simulink model "Aim_23__Monocopter_Testing"  (R2023b)
settings: Solver=ode23t  StartTime=0.0  StopTime=10  MaxStep=1e-3  RelTol=1e-3  AbsTol=1e-3
values from neighbouring files (symbols this model uses):
  air_rho = 1.225    [Aim_23_inherited_params.mat]
  battery_capacity = 22.8    [Aim_23_inherited_params.mat]
  CDO = 10.25    [Aim_23_inherited_params.mat]
  drag_linear = 0.002    [Aim_23_inherited_params.mat]
  drag_quad = 0.005    [Aim_23_inherited_params.mat]
  filtD_motor = 100    [Aim_23_inherited_params.mat]
  filtSpd_motor = 0.001    [Aim_23_inherited_params.mat]
  flap_radius = 0.05312    [Aim_23_inherited_params.mat]
  flap_surface_area = 0.025    [Aim_23_inherited_params.mat]
  kd_motor = 0    [Aim_23_inherited_params.mat]
  ki_motor = 0.00045    [Aim_23_inherited_params.mat]
  klinear = 0.03    [Aim_23_inherited_params.mat]
  kquad = 0.025    [Aim_23_inherited_params.mat]
  limit_motor = 0.25    [Aim_23_inherited_params.mat]
  monoco_mass = 160    [Aim_23_inherited_params.mat]
  monoco_prop =     [Aim_23_inherited_params.mat]
  monoco_radius = 0.61    [Aim_23_inherited_params.mat]
  monoco_wing =     [Aim_23_inherited_params.mat]
  monoco_wing_area = 0.239    [Aim_23_inherited_params.mat]
  waypoints = [-2 -2 0.14 -2 -2 6 0 0 6 2 0 6 ... (15 elements, 3x5)]    [Aim_23_inherited_params.mat]
undefined symbols (not defined in the file or in its folder): X, Y, Z
libraries: sm_lib x97, nesl_utility x38, slpidlib x18, fl_lib x12, sdl_lib x3, simulink x2, simulink_extras x1, batteryecm_lib x1, ee_lib x1
(part 2 of 7)

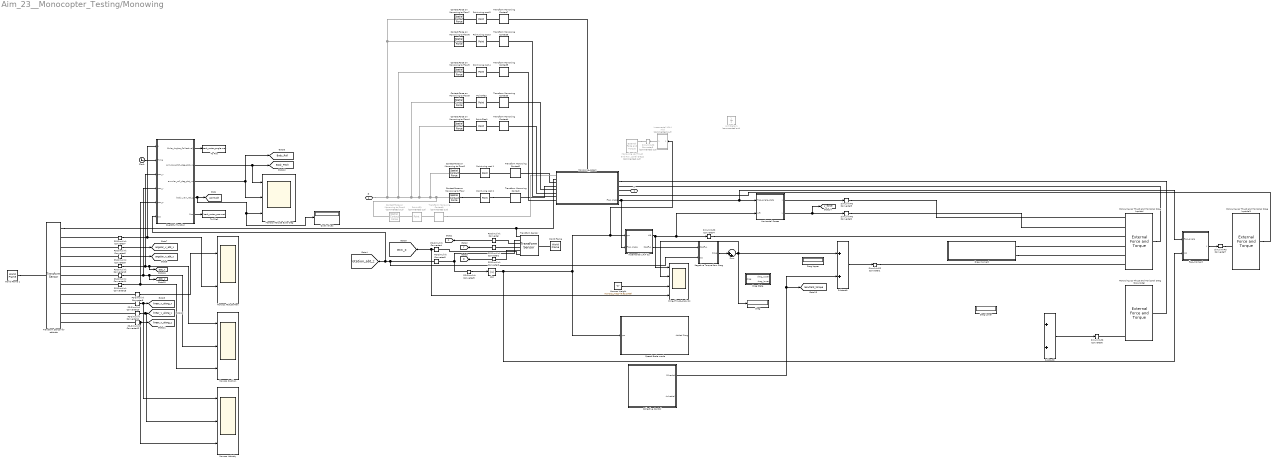
== system Aim_23__Monocopter_Testing/Monowing ==
  Abs : Abs  SaturateOnIntegerOverflow=off
  Clock : Clock
  Collective Control : Subsystem
  Contact Force on Monowing to Floor{,2..7} (7 alike) : sm_lib/Forces and Torques/Spatial Contact Force  SenseContactBaseRotation=off  SenseContactBaseTranslation=off  CoefficientOfDynamicFriction=0  CoefficientOfStaticFriction=0  NormalDamping=pkgGrndDamp  NormalDampingUnits=N/(m/s)  SenseContactSignal=off  NormalStiffness=pkgGrndStiff  NormalStiffnessUnits=N/m  FrictionalCriticalVelocity=1e-2  FrictionalCriticalVelocityUnits=m/s  ZeroCrossDetectContactStartAndEnd=off  SenseContactFollowerRotation=off  SenseContactFollowerTranslation=off  FrictionType=SmoothStickSlip  SenseFrictionalForceMagnitude=off  SenseNormalForceMagnitude=off  NormalForceType=SmoothSpringDamper  SenseNormalVelocity=off  SensePenetrationDepth=off  SenseSeparationDistance=off  SenseTangentialVelocity=off  NormalTransitionRegionWidth=pkgGrndTransW  NormalTransitionRegionWidthUnits=m
  Contact Force on Monowing to Floor1 : sm_lib/Forces and Torques/Spatial Contact Force  Commented=on  SenseContactBaseRotation=off  SenseContactBaseTranslation=off  CoefficientOfDynamicFriction=0  CoefficientOfStaticFriction=0  NormalDamping=pkgGrndDamp  NormalDampingUnits=N/(m/s)  SenseContactSignal=off  NormalStiffness=pkgGrndStiff  NormalStiffnessUnits=N/m  FrictionalCriticalVelocity=1e-2  FrictionalCriticalVelocityUnits=m/s  ZeroCrossDetectContactStartAndEnd=off  SenseContactFollowerRotation=off  SenseContactFollowerTranslation=off  FrictionType=SmoothStickSlip  SenseFrictionalForceMagnitude=off  SenseNormalForceMagnitude=off  NormalForceType=SmoothSpringDamper  SenseNormalVelocity=off  SensePenetrationDepth=off  SenseSeparationDistance=off  SenseTangentialVelocity=off  NormalTransitionRegionWidth=pkgGrndTransW  NormalTransitionRegionWidthUnits=m
  Drag : Display
  Drag Lower : Display
  Drag State : Subsystem
  Drag Upper : Display
  Drag moment : Subsystem
  Horizontal Forces : Subsystem
  Incremental Lift 4 mid : Subsystem  Commented=on
  Incremental Lift 4 tip : Subsystem
  Monoco Attitude Euler Deg : Scope  NumInputPorts=3
  Monoco Attitude Raw : Scope  NumInputPorts=2
  Monoco Position : Scope  NumInputPorts=3
  Monoco Velocity : Scope  NumInputPorts=3
  Monoco Weight : Constant  Value=monoco_mass*(9.81/1000)
  Monowing Up Thrust and Horizonal Drag (Downside) : sm_lib/Forces and Torques/External Force and Torque  ForceResolutionFrame=World  EnableForceX=on  EnableForceY=on  EnableForceZ=on  EnableForce=off  TorqueResolutionFrame=World  EnableTorqueX=on  EnableTorqueY=on  EnableTorqueZ=on  EnableTorque=off
  Monowing Up Thrust and Horizonal Drag (upside) : sm_lib/Forces and Torques/External Force and Torque  ForceResolutionFrame=World  EnableForceX=on  EnableForceY=on  EnableForceZ=on  EnableForce=off  TorqueResolutionFrame=World  EnableTorqueX=on  EnableTorqueY=on  EnableTorqueZ=on  EnableTorque=off
  Monowing Up Thrust and Horizonal Drag (upside)1 : sm_lib/Forces and Torques/External Force and Torque  ForceResolutionFrame=World  EnableForceX=on  EnableForceY=on  EnableForceZ=on  EnableForce=off  TorqueResolutionFrame=World  EnableTorqueX=on  EnableTorqueY=on  EnableTorqueZ=on  EnableTorque=off
  Monowing Up Thrust and Horizonal Drag2 : sm_lib/Forces and Torques/External Force and Torque  Commented=on  ForceResolutionFrame=World  EnableForceX=off  EnableForceY=off  EnableForceZ=on  EnableForce=off  TorqueResolutionFrame=World  EnableTorqueX=on  EnableTorqueY=off  EnableTorqueZ=on  EnableTorque=off
  Monowing_Assem : Subsystem
      settings: PortSchema="{\"entries\":[{\"content\":{\"sides\":[{\"content\":{\"connectorIds\":[\"LConn1\",\"LConn2\",\"LConn3\",\"LConn4\",\"LConn5\",\"Out1\"]},\"type\":\"ConnectorPlacement.EquallySpacedRectSide\",\"uuid\":\"ac7a8aa6-e60b-47ca-89e5-d63ad1015c78\"},{\"content\":{\"connectorIds\":[\"RConn1\",\"RConn2\",\"RConn3\",\"RConn4\",\"RConn5\",\"RConn6\",\"RConn7\",\"RConn8\"],\"side\":\"RIGHT\"},\"type\":\"ConnectorPlacement.EquallySpacedRectSide\",\"uuid\":\"7d8b3f85-eefd-43b2-ace0-dcd753a78691\"},{\"content\":{\"connectorIds\":[\"LConn6\"],\"side\":\"TOP\"},\"type\":\"ConnectorPlacement.EquallySpacedRectSide\",\"uuid\":\"e2e303e2-d724-4fc3-8dfb-5b8cdd8963e9\"}]},\"type\":\"ConnectorPlacement.EquallySpacedConnector\",\"uuid\":\"fd6e9b64-e855-43fb-9cb5-0f36294065cb\"}],\"packageUris\":[\"http://schema.mathworks.com/mf0/Connector/R2020b\"],\"version\":\"1.0\"}"
  Negative Torque from Drag : Subsystem
  PS-Simulink Converter{,1..2,4..6,8..15} (14 alike) : nesl_utility/PS-Simulink Converter  PhysicalDomain=network_engine_domain  SubClassName=ps_output  LeftPortType=input  RightPortType=output  PseudoPeriodic=off  Frequencies=[]  VectorFormat=inherit  Unit=inherit  AffineConversion=off
  PS-Simulink Converter3 : nesl_utility/PS-Simulink Converter  PhysicalDomain=network_engine_domain  SubClassName=ps_output  LeftPortType=input  RightPortType=output  PseudoPeriodic=off  Frequencies=[]  VectorFormat=1-D array  Unit=inherit  AffineConversion=off
  PS-Simulink Converter7 : nesl_utility/PS-Simulink Converter  PhysicalDomain=network_engine_domain  SubClassName=ps_output  LeftPortType=input  RightPortType=output  PseudoPeriodic=off  Frequencies=[]  VectorFormat=1-D array  Unit=inherit  AffineConversion=off
  Point Flap : sm_lib/Curves and Surfaces/Point  GraphicType=Marker  MarkerShape=Cube  MarkerSize=20  GraphicVisPropType=SimpleVisualProperties  GraphicDiffuseColor=[0.5 0.5 0.5]  GraphicOpacity=0  GraphicSpecularColor=[0.5 0.5 0.5 1.0]  GraphicAmbientColor=[0.15 0.15 0.15 1.0]  GraphicEmissiveColor=[0.0 0.0 0.0 1.0]  GraphicShininess=75
  Point Flap1 : sm_lib/Curves and Surfaces/Point  GraphicType=Marker  MarkerShape=Cube  MarkerSize=20  GraphicVisPropType=SimpleVisualProperties  GraphicDiffuseColor=[0.5 0.5 0.5]  GraphicOpacity=0  GraphicSpecularColor=[0.5 0.5 0.5 1.0]  GraphicAmbientColor=[0.15 0.15 0.15 1.0]  GraphicEmissiveColor=[0.0 0.0 0.0 1.0]  GraphicShininess=75
  Point LR1 : sm_lib/Curves and Surfaces/Point  Commented=on  GraphicType=Marker  MarkerShape=Frame  MarkerSize=100  GraphicVisPropType=SimpleVisualProperties  GraphicDiffuseColor=[0.5 0.5 0.5]  GraphicOpacity=0  GraphicSpecularColor=[0.5 0.5 0.5 1.0]  GraphicAmbientColor=[0.15 0.15 0.15 1.0]  GraphicEmissiveColor=[0.0 0.0 0.0 1.0]  GraphicShininess=75
  Point wing root {1..5} (5 alike) : sm_lib/Curves and Surfaces/Point  GraphicType=Marker  MarkerShape=Cube  MarkerSize=20  GraphicVisPropType=SimpleVisualProperties  GraphicDiffuseColor=[0.5 0.5 0.5]  GraphicOpacity=0  GraphicSpecularColor=[0.5 0.5 0.5 1.0]  GraphicAmbientColor=[0.15 0.15 0.15 1.0]  GraphicEmissiveColor=[0.0 0.0 0.0 1.0]  GraphicShininess=75
  Quat values : Display
  Quat2Eul Function : MATLAB Function  TreatAsAtomicUnit=on
  Simulink-PS Converter{1..4,6..7} (6 alike) : nesl_utility/Simulink-PS Converter  PhysicalDomain=network_engine_domain  SubClassName=ps_input  LeftPortType=input  RightPortType=output  PseudoPeriodic=off  Frequencies=[]  NoiseDistribution=none  NoiseParameters=[]  Unit=1  AffineConversion=off  FilteringAndDerivatives=provide  SimscapeFilterOrder=1  InputFilterTimeConstant=0.001  UdotUserProvided=0
  Simulink-PS Converter5 : nesl_utility/Simulink-PS Converter  Commented=on  PhysicalDomain=network_engine_domain  SubClassName=ps_input  LeftPortType=input  RightPortType=output  PseudoPeriodic=off  Frequencies=[]  NoiseDistribution=none  NoiseParameters=[]  Unit=1  AffineConversion=off  FilteringAndDerivatives=provide  SimscapeFilterOrder=1  InputFilterTimeConstant=0.001  UdotUserProvided=0
  Speed Brake mode : Subsystem
  Subtract1 : Sum
  Subtract2 : Sum
  Sum : Sum  Inputs=|++
  To File : ToFile  Filename=back_motor_angle.mat  MatrixName=txyzangle
  To File1 : ToFile  Filename=back_motor_pos.mat  MatrixName=txyzposrps
  Transform Monowing Contact : sm_lib/Frames and Transforms/Rigid Transform  TranslationMethod=Cartesian  TranslationStandardOffset=0.08  TranslationStandardOffsetUnits=mm  TranslationStandardAxis=-Y  TranslationCartesianOffset=[107 -50 -6]  TranslationCartesianOffsetUnits=mm  TranslationROffset=0  TranslationROffsetUnits=m  TranslationZOffset=0  TranslationZOffsetUnits=m  TranslationThetaOffset=0  TranslationThetaOffsetUnits=deg  RotationMethod=None  RotationAngleUnits=deg  RotationStandardAxis=+X  RotationAngle=90  RotationArbitraryAxis=[0 0 1]  FollAlignAxisA=+X  BaseAlignAxisA=+Y  FollAlignAxisB=+Y  BaseAlignAxisB=+Z  RotationSequenceAxes=FollowerAxes  RotationSequence=XYX  RotationSequenceAngles=[0 0 0]  RotationSequenceAnglesUnits=deg  RotationMatrix=[1 0 0; 0 1 0; 0 0 1]  Quaternion=[1 0 0 0]
  Transform Monowing Contact1 : sm_lib/Frames and Transforms/Rigid Transform  Commented=on  TranslationMethod=Cartesian  TranslationStandardOffset=0.08  TranslationStandardOffsetUnits=m  TranslationStandardAxis=-Y  TranslationCartesianOffset=[0 0 0]  TranslationCartesianOffsetUnits=m  TranslationROffset=0  TranslationROffsetUnits=m  TranslationZOffset=0  TranslationZOffsetUnits=m  TranslationThetaOffset=0  TranslationThetaOffsetUnits=deg  RotationMethod=None  RotationAngleUnits=deg  RotationStandardAxis=+X  RotationAngle=90  RotationArbitraryAxis=[0 0 1]  FollAlignAxisA=+X  BaseAlignAxisA=+Y  FollAlignAxisB=+Y  BaseAlignAxisB=+Z  RotationSequenceAxes=FollowerAxes  RotationSequence=XYX  RotationSequenceAngles=[0 0 0]  RotationSequenceAnglesUnits=deg  RotationMatrix=[1 0 0; 0 1 0; 0 0 1]  Quaternion=[1 0 0 0]
  Transform Monowing Contact2 : sm_lib/Frames and Transforms/Rigid Transform  TranslationMethod=Cartesian  TranslationStandardOffset=0.08  TranslationStandardOffsetUnits=mm  TranslationStandardAxis=-Y  TranslationCartesianOffset=[107 -10 -6]  TranslationCartesianOffsetUnits=mm  TranslationROffset=0  TranslationROffsetUnits=m  TranslationZOffset=0  TranslationZOffsetUnits=m  TranslationThetaOffset=0  TranslationThetaOffsetUnits=deg  RotationMethod=None  RotationAngleUnits=deg  RotationStandardAxis=+X  RotationAngle=90  RotationArbitraryAxis=[0 0 1]  FollAlignAxisA=+X  BaseAlignAxisA=+Y  FollAlignAxisB=+Y  BaseAlignAxisB=+Z  RotationSequenceAxes=FollowerAxes  RotationSequence=XYX  RotationSequenceAngles=[0 0 0]  RotationSequenceAnglesUnits=deg  RotationMatrix=[1 0 0; 0 1 0; 0 0 1]  Quaternion=[1 0 0 0]
  Transform Monowing Contact{3..7} (5 alike) : sm_lib/Frames and Transforms/Rigid Transform  TranslationMethod=Cartesian  TranslationStandardOffset=0.08  TranslationStandardOffsetUnits=mm  TranslationStandardAxis=-Y  TranslationCartesianOffset=[0 0 0]  TranslationCartesianOffsetUnits=mm  TranslationROffset=0  TranslationROffsetUnits=m  TranslationZOffset=0  TranslationZOffsetUnits=m  TranslationThetaOffset=0  TranslationThetaOffsetUnits=deg  RotationMethod=None  RotationAngleUnits=deg  RotationStandardAxis=+X  RotationAngle=90  RotationArbitraryAxis=[0 0 1]  FollAlignAxisA=+X  BaseAlignAxisA=+Y  FollAlignAxisB=+Y  BaseAlignAxisB=+Z  RotationSequenceAxes=FollowerAxes  RotationSequence=XYX  RotationSequenceAngles=[0 0 0]  RotationSequenceAnglesUnits=deg  RotationMatrix=[1 0 0; 0 1 0; 0 0 1]  Quaternion=[1 0 0 0]
  Transform Sensor : sm_lib/Frames and Transforms/Transform Sensor  MeasurementFrame=World  RotationSequence=XYX  SenseAngle=off  SenseAxis=off  SenseQ=off  SenseR=off  SenseRotationSequence=off  SenseOmegaX=off  SenseOmegaY=off  SenseOmegaZ=on  SenseOmega=off  SenseQDot=off  SenseRDot=off  SenseRotationSequenceDot=off  SenseAlphaX=off  SenseAlphaY=off  SenseAlphaZ=off  SenseAlpha=off  SenseQDDot=off  SenseRDDot=off  SenseX=on  SenseY=on  SenseZ=on  SenseXYZ=off  SenseRad=off  SenseAzim=off  SenseDist=off  SenseInc=off  SenseXDot=off  SenseYDot=off  SenseZDot=off  SenseXYZDot=off  SenseRadDot=off  SenseAzimDot=off  SenseDistDot=off  SenseIncDot=off  SenseXDDot=off  SenseYDDot=off  SenseZDDot=on  SenseXYZDDot=off  SenseRadDDot=off  SenseAzimDDot=off  SenseDistDDot=off  SenseIncDDot=off
  Transform Sensor for attitude : sm_lib/Frames and Transforms/Transform Sensor  MeasurementFrame=World  RotationSequence=XYX  SenseAngle=off  SenseAxis=off  SenseQ=on  SenseR=off  SenseRotationSequence=off  SenseOmegaX=on  SenseOmegaY=on  SenseOmegaZ=off  SenseOmega=off  SenseQDot=off  SenseRDot=off  SenseRotationSequenceDot=off  SenseAlphaX=off  SenseAlphaY=off  SenseAlphaZ=off  SenseAlpha=off  SenseQDDot=off  SenseRDDot=off  SenseX=on  SenseY=on  SenseZ=on  SenseXYZ=off  SenseRad=off  SenseAzim=on  SenseDist=off  SenseInc=off  SenseXDot=on  SenseYDot=on  SenseZDot=on  SenseXYZDot=off  SenseRadDot=off  SenseAzimDot=off  SenseDistDot=off  SenseIncDot=off  SenseXDDot=off  SenseYDDot=off  SenseZDDot=off  SenseXYZDDot=off  SenseRadDDot=off  SenseAzimDDot=off  SenseDistDDot=off  SenseIncDDot=off
  Unit Delay1 : UnitDelay  Commented=on  HasFrameUpgradeWarning=on
  Wing_Thrust_Analysis : Scope  NumInputPorts=4
  World Frame : sm_lib/Frames and Transforms/World Frame
  World Frame 1 : sm_lib/Frames and Transforms/World Frame
  "flap_moment " : MATLAB Function  TreatAsAtomicUnit=on
  M : PMIOPort  Side=Left
  G : PMIOPort  Port=2  Side=Right
  tag scope: Azimuth=global, Body_Pitch=global, Body_Roll=global, X=global, Y=global, Z=global, acc_z=global, angular_v_abt_x=global, angular_v_abt_y=global, linear_v_along_x=global, linear_v_along_y=global, linear_v_along_z=global, pos_x=global, pos_y=global, resultant_torque=global, rotation_abt_z=global, y_force=global
  wires:
  PS-Simulink Converter1/1 -> [Y]
  PS-Simulink Converter/1 -> [X]
  PS-Simulink Converter2/1 -> [Z]
  PS-Simulink Converter3/1 -> Quat2Eul Function/6(rps), [rotation_abt_z], Negative Torque from Drag/2(rps)
  Monoco Weight/1 -> Wing_Thrust_Analysis/3
  Abs/1 -> "flap_moment "/2(rps), Speed Brake mode/1(rps), Incremental Lift 4 tip/1(rps), Incremental Lift 4 mid/1(In1)
  PS-Simulink Converter4/1 -> Wing_Thrust_Analysis/4, [acc_z]
  Incremental Lift 4 tip/1(Lift) -> Horizontal Forces/2(Lift), Simulink-PS Converter4/1, Wing_Thrust_Analysis/1
  Incremental Lift 4 mid/1(Out1) -> Simulink-PS Converter5/1
  Negative Torque from Drag/1(Drag) -> Sum/1
  Subtract1/1 -> Simulink-PS Converter1/1
  PS-Simulink Converter7/1 -> Monoco Attitude Raw/2, Quat2Eul Function/1(u)
  Quat2Eul Function/2(annular_pitch_deg_abt_yw) -> Monoco Attitude Euler Deg/1, [Body_Pitch]
  Quat2Eul Function/4(body_yaw_rad_z) -> Quat values/1, Monoco Attitude Euler Deg/3, [Azimuth]
  Monowing_Assem/1(Flap Angle) -> "flap_moment "/1(flap_angle), Horizontal Forces/1(flap_angle_data), Incremental Lift 4 tip/2(Flap Angle)
  Incremental Lift 4 tip/2(Coeff_L) -> Negative Torque from Drag/1(Coeff_L)
  PS-Simulink Converter6/1 -> [angular_v_abt_x]
  PS-Simulink Converter9/1 -> [angular_v_abt_y]
  Quat2Eul Function/1(Euler_Angles_Collectively) -> To File/1
  PS-Simulink Converter10/1 -> Monoco Velocity/1, [linear_v_along_x]
  PS-Simulink Converter11/1 -> [linear_v_along_y], Monoco Velocity/2
  PS-Simulink Converter12/1 -> Monoco Velocity/3, [linear_v_along_z]
  PS-Simulink Converter8/1 -> Monoco Attitude Raw/1
  PS-Simulink Converter13/1 -> Quat2Eul Function/3(pos_x), [pos_x], Monoco Position/1
  PS-Simulink Converter14/1 -> Quat2Eul Function/4(pos_y), [pos_y], Monoco Position/2
  PS-Simulink Converter15/1 -> Quat2Eul Function/5(pos_z), Monoco Position/3
  Quat2Eul Function/3(annular_roll_deg_abt_xw) -> Monoco Attitude Euler Deg/2, [Body_Roll]
  Horizontal Forces/2(y) -> [y_force], Simulink-PS Converter2/1
  PS-Simulink Converter5/1 -> Abs/1
  Sum/1 -> Drag/1, Subtract1/1, Wing_Thrust_Analysis/2
  Subtract2/1 -> Simulink-PS Converter6/1
  Collective Control/1(Dihedral) -> Subtract1/2, [resultant_torque]
  Horizontal Forces/1(x) -> Simulink-PS Converter3/1
  "flap_moment "/1(y) -> Simulink-PS Converter7/1
  Clock/1 -> Quat2Eul Function/2(Time)
  Quat2Eul Function/5(Pos) -> To File1/1
  connections:
  World Frame/RConn1 -- Transform Sensor/LConn1
  Point wing root 2/LConn1 -- Transform Monowing Contact/RConn1
  Contact Force on Monowing to Floor/LConn1 -- Point wing root 2/RConn1
  Contact Force on Monowing to Floor1/RConn1 -- Contact Force on Monowing to Floor4/RConn1 -- Contact Force on Monowing to Floor7/RConn1 -- Contact Force on Monowing to Floor6/RConn1 -- G/RConn1 -- Contact Force on Monowing to Floor5/RConn1 -- Contact Force on Monowing to Floor3/RConn1 -- Contact Force on Monowing to Floor2/RConn1 -- Contact Force on Monowing to Floor/RConn1
  Transform Monowing Contact1/RConn1 -- Point LR1/LConn1
  Point LR1/RConn1 -- Contact Force on Monowing to Floor1/LConn1
  Transform Sensor/RConn3 -- PS-Simulink Converter/LConn1
  Transform Sensor/RConn4 -- PS-Simulink Converter1/LConn1
  Transform Sensor/RConn5 -- PS-Simulink Converter2/LConn1
  Transform Sensor/RConn2 -- PS-Simulink Converter5/LConn1 -- PS-Simulink Converter3/LConn1
  M/RConn1 -- Monowing_Assem/LConn4
  Monowing_Assem/RConn2 -- Transform Sensor/RConn1 -- Transform Sensor for attitude/RConn1
  Transform Monowing Contact2/RConn1 -- Point wing root 1/LConn1
  Point wing root 1/RConn1 -- Contact Force on Monowing to Floor2/LConn1
  Monowing_Assem/RConn3 -- Transform Monowing Contact2/LConn1
  Monowing_Assem/RConn4 -- Transform Monowing Contact/LConn1
  Transform Monowing Contact1/LConn1 -- Monowing_Assem/RConn1
  Transform Sensor/RConn6 -- PS-Simulink Converter4/LConn1
  Monowing Up Thrust and Horizonal Drag (upside)/RConn1 -- Monowing_Assem/LConn3
  Monowing Up Thrust and Horizonal Drag2/LConn1 -- Simulink-PS Converter5/RConn1
  World Frame 1/RConn1 -- Transform Sensor for attitude/LConn1
  PS-Simulink Converter7/LConn1 -- Transform Sensor for attitude/RConn2
  PS-Simulink Converter6/LConn1 -- Transform Sensor for attitude/RConn3
  PS-Simulink Converter9/LConn1 -- Transform Sensor for attitude/RConn4
  PS-Simulink Converter12/LConn1 -- Transform Sensor for attitude/RConn11
  PS-Simulink Converter11/LConn1 -- Transform Sensor for attitude/RConn10
  PS-Simulink Converter10/LConn1 -- Transform Sensor for attitude/RConn9
  PS-Simulink Converter8/LConn1 -- Transform Sensor for attitude/RConn8
  PS-Simulink Converter13/LConn1 -- Transform Sensor for attitude/RConn5
  PS-Simulink Converter14/LConn1 -- Transform Sensor for attitude/RConn6
  PS-Simulink Converter15/LConn1 -- Transform Sensor for attitude/RConn7
  Monowing_Assem/LConn2 -- Monowing Up Thrust and Horizonal Drag (Downside)/RConn1
  Simulink-PS Converter1/RConn1 -- Monowing Up Thrust and Horizonal Drag (upside)/LConn6
  Monowing Up Thrust and Horizonal Drag (Downside)/LConn6 -- Simulink-PS Converter6/RConn1
  Transform Monowing Contact3/RConn1 -- Point Flap/LConn1
  Point Flap/RConn1 -- Contact Force on Monowing to Floor3/LConn1
  Monowing_Assem/RConn5 -- Transform Monowing Contact3/LConn1
  Transform Monowing Contact4/RConn1 -- Point Flap1/LConn1
  Point Flap1/RConn1 -- Contact Force on Monowing to Floor4/LConn1
  Monowing_Assem/RConn6 -- Transform Monowing Contact4/LConn1
  Transform Monowing Contact5/RConn1 -- Point wing root 4/LConn1
  Point wing root 4/RConn1 -- Contact Force on Monowing to Floor5/LConn1
  Transform Monowing Contact6/RConn1 -- Point wing root 3/LConn1
  Point wing root 3/RConn1 -- Contact Force on Monowing to Floor6/LConn1
  Monowing_Assem/RConn7 -- Transform Monowing Contact6/LConn1
  Monowing_Assem/RConn8 -- Transform Monowing Contact5/LConn1
  Point wing root 5/RConn1 -- Contact Force on Monowing to Floor7/LConn1
  Transform Monowing Contact7/RConn1 -- Point wing root 5/LConn1
  Monowing_Assem/LConn6 -- Transform Monowing Contact7/LConn1
  Simulink-PS Converter2/RConn1 -- Monowing Up Thrust and Horizonal Drag (upside)/LConn2
  Simulink-PS Converter3/RConn1 -- Monowing Up Thrust and Horizonal Drag (upside)/LConn1
  Drag moment/RConn1 -- Monowing Up Thrust and Horizonal Drag (upside)/LConn4
  Drag moment/RConn2 -- Monowing Up Thrust and Horizonal Drag (upside)/LConn5
  Simulink-PS Converter4/RConn1 -- Monowing Up Thrust and Horizonal Drag (upside)/LConn3
  Monowing Up Thrust and Horizonal Drag (upside)1/RConn1 -- Monowing_Assem/LConn5
  Simulink-PS Converter7/RConn1 -- Monowing Up Thrust and Horizonal Drag (upside)1/LConn4

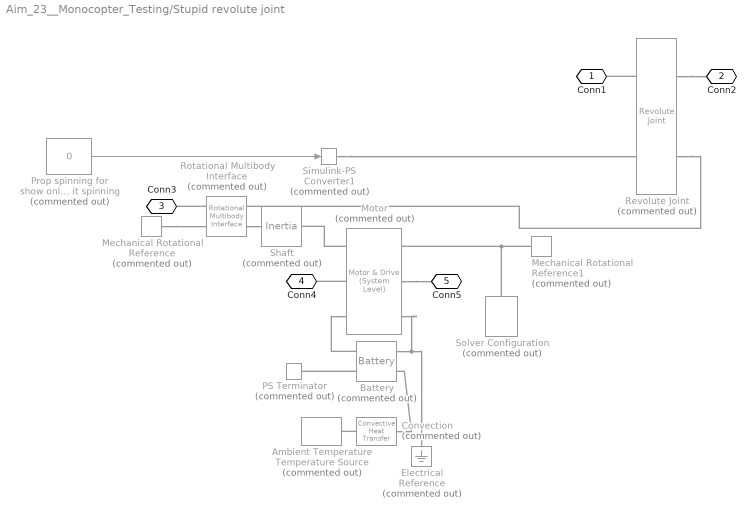
== system Aim_23__Monocopter_Testing/Stupid revolute joint ==
  Ambient Temperature : fl_lib/Thermal/Thermal Sources/Temperature Source  Commented=on  temperature=air_temperature K
  Battery : batteryecm_lib/Battery  Commented=on  Vnom=14 V  prm_dir=1  R1_dis=2 Ohm  R1_ch=2 Ohm  R1=2e-2 Ohm  prm_AH=2  AH=battery_capacity A*hr  V1=11.5 V  AH1=battery_capacity/2 A*hr  prm_R2=1  R2=2000 Ohm  prm_dyn=1  Rp1=0.005 Ohm  tau1=30 s  Rp2=0.005 Ohm  tau2=30 s  Rp3=0.005 Ohm  tau3=30 s  Rp4=0.005 Ohm  tau4=30 s  Rp5=0.005 Ohm  tau5=30 s  prm_fade=1  N_fade=100  AH_fade=45 A*hr  R1_fade=2.02 Ohm  R1_ch_fade=2.02 Ohm  V1_fade=10.35 V  prm_age=1  prm_age_OCV=1  OCV_age=0.9  SOC_age=60  delta_time_age_vec=[0] d  temperature_age_vec=[273] K  OCV_scaling_age=2.2134e6  OCV_offset_age=1.632e6  temp_exp_age=0.515833569 V  t_exp_age=0.75  i_specify=off  i_priority=None  i=0 A  i_nominal_specify=off  i_nominal_unit=A  i_nominal_value=1  v_specify=off  v_priority=None  v=0 V  v_nominal_specify=off  v_nominal_unit=V  v_nominal_value=1  charge_specify=on  charge_priority=High  charge=battery_capacity A*hr  charge_nominal_specify=off  charge_nominal_unit=A*hr  charge_nominal_value=1  num_cycles_specify=off  num_cycles_priority=High  num_cycles=0  num_cycles_nominal_specify=off  num_cycles_nominal_unit=1  num_cycles_nominal_value=1  Tmeas=298.15 K  Tmeas_age=298.15 K  Vnom_T2=12 V  R1_T2=2e-2 Ohm  R1_T2_dis=2.2 Ohm  R1_T2_ch=2.2 Ohm  V1_T2=11.4 V  R2_T2=2200 Ohm  Rp1_T2=0.005 Ohm  tau1_T2=30 s  Rp2_T2=0.005 Ohm  tau2_T2=30 s  Rp3_T2=0.005 Ohm  tau3_T2=30 s  Rp4_T2=0.005 Ohm  tau4_T2=30 s  Rp5_T2=0.005 Ohm  tau5_T2=30 s  Tmeas2=273.15 K  thermal_mass=30000 J/K  temperature_specify=on  temperature_priority=High  temperature=air_temperature K  temperature_nominal_specify=off  temperature_nominal_unit=K  temperature_nominal_value=1
      settings: InternalSimscapePortConfiguration="{\"Bottom\":[],\"Left\":[{\"id\":\"p\",\"label\":\"+\",\"type\":\"foundation.electrical.electrical\"},{\"id\":\"q\",\"label\":\"q\",\"type\":\"output\"}],\"Right\":[{\"id\":\"n\",\"label\":\"-\",\"type\":\"foundation.electrical.electrical\"},{\"id\":\"H\",\"label\":\"H\",\"type\":\"foundation.thermal.thermal\"}],\"Top\":[]}"
  Convection : fl_lib/Thermal/Thermal Elements/Convective Heat Transfer  Commented=on  thermal_type=foundation.enum.constant_variable.constant  area=3e-3 m^2  heat_tr_coeff=20 W/(m^2*K)  min_heat_tr_coeff=1e-3 W/(K*m^2)  T_specify=off  T_priority=None  T=0 K  T_nominal_specify=off  T_nominal_unit=K  T_nominal_value=1  Q_specify=off  Q_priority=None  Q=0 W  Q_nominal_specify=off  Q_nominal_unit=W  Q_nominal_value=1
  Electrical Reference : fl_lib/Electrical/Electrical Elements/Electrical Reference  Commented=on
  Mechanical Rotational Reference : fl_lib/Mechanical/Rotational Elements/Mechanical Rotational Reference  Commented=on
  Mechanical Rotational Reference1 : fl_lib/Mechanical/Rotational Elements/Mechanical Rotational Reference  Commented=on
  Motor : ee_lib/Electromechanical/Motor & Drive (System Level)  Commented=on  torque_speed_param=ee.enum.electromech.envelope.torque_power  overtorque_param=ee.enum.electromech.overtorque.no  T_t=[.09, .08, .07, 0] N*m  T_t_intermittent=[.36, .32, .28, 0] N*m  T_t_2D=[.09, .09, .09; .08, .08, .08; .07, .07, .07; 0, 0, 0] N*m  T_t_intermittent_2D=[.36, .36, .36; .32, .32, .32; .28, .28, .28; 0, 0, 0] N*m  w_t=[0, 3750, 7500, 8000] rpm  vdc_t=[6, 12, 24] V  torque_max=qc_motor.max_torque N*m  power_max=motor_max_power W  torque_max_intermittent=0.4 N*m  power_max_intermittent=120 W  time_overtorque=30 s  time_recover=60 s  Tc=qc_motor.time_const s  losses_param=1  eff=qc_motor.efficiency  w_eff=qc_motor.efficiency_spd rpm  T_eff=qc_motor.efficiency_trq N*m  Piron=0 W  Pbase="0  W"  w_eff_vec=[-8000, -4000, 0, 4000, 8000] rpm  T_eff_vec=[0, .03, .06, .09] N*m  v_eff_vec=[100, 250, 400] V  losses_mat=[1.49, 1.67, 2.21, 3.1; .42, .69, 1.14, 2.03; .06, .24, .78, 1.68; .42, .69, 1.14, 2.03; 1.49, 1.67, 2.21, 3.1] W  efficiency_mat=[95, 95, 95, 95; 95, 95, 95, 95; 95, 95, 95, 95; 95, 95, 95, 95; 95, 95, 95, 95]  losses_mat_3D=ones(5, 4, 3) W  efficiency_mat_3D=95 * ones(5, 4, 3)  Res="0  Ohm"  enable_fault=simscape.enum.onoff.off  fault_condition=1  fault_threshold=0.5  J=0 kg*m^2  lam=qc_motor.rotor_damping N*m/(rad/s)  speed0=0 rpm  faulted_specify=off  faulted_priority=None  faulted=0  faulted_nominal_specify=off  faulted_nominal_unit=1  faulted_nominal_value=1  torqueLimitContinuous_specify=off  torqueLimitContinuous_priority=None  torqueLimitContinuous=0 N*m  torqueLimitContinuous_nominal_specify=off  torqueLimitContinuous_nominal_unit=N*m  torqueLimitContinuous_nominal_value=1  alpha=3.93e-3 1/K  Tmeas=25 degC  Tmeas2=125 degC  losses_mat_T2=[1.49, 1.74, 2.49, 3.74; .42, .67, 1.42, 2.67; .06, .31, 1.06, 2.31; .42, .67, 1.42, 2.67; 1.49, 1.74, 2.49, 3.74] W  efficiency_mat_T2=[95, 95, 95, 95; 95, 95, 95, 95; 95, 95, 95, 95; 95, 95, 95, 95; 95, 95, 95, 95]  losses_mat_3D_T2=ones(5, 4, 3) W  efficiency_mat_3D_T2=95 * ones(5, 4, 3)  thermal_mass=100 J/K  initial_temperature=25 degC
  PS Terminator : fl_lib/Physical Signals/Sinks/PS Terminator  Commented=on
  "Prop spinning for show only LOL, put -0.0003 to show it spinning" : Constant  Commented=on  Value=0
  Revolute Joint : sm_lib/Joints/Revolute Joint  Commented=on  JointMode=Normal  SenseConstraintForce=off  SenseConstraintForceX=off  SenseConstraintForceY=off  SenseConstraintForceZ=off  SenseConstraintTorque=off  SenseConstraintTorqueX=off  SenseConstraintTorqueY=off  SenseConstraintTorqueZ=off  SenseTotalForce=off  SenseTotalForceX=off  SenseTotalForceY=off  SenseTotalForceZ=off  SenseTotalTorque=off  SenseTotalTorqueX=off  SenseTotalTorqueY=off  SenseTotalTorqueZ=off  CompositeWrenchDir=FollowerOnBase  CompositeWrenchFrame=BaseFrame  EquilibriumPosition=0  EquilibriumPositionUnits=deg  SpringStiffness=0  SpringStiffnessUnits=N*m/rad  DampingCoefficient=1e-5  DampingCoefficientUnits=N*m/(rad/s)  TorqueActuationMode=InputTorque  MotionActuationMode=ComputedMotion  SensePosition=off  SenseVelocity=on  SenseAcceleration=off  SenseTorqueForce=off  SenseLowerLimitTorqueForce=off  SenseUpperLimitTorqueForce=off  LowerLimitSpecify=off  LowerLimitBound=-90  LowerLimitBoundUnits=deg  LowerLimitStiffness=1e4  LowerLimitStiffnessUnits=N*m/deg  LowerLimitDamping=10  LowerLimitDampingUnits=N*m/(deg/s)  LowerLimitTransitionRegionWidth=0.1  LowerLimitTransitionRegionWidthUnits=deg  UpperLimitSpecify=off  UpperLimitBound=90  UpperLimitBoundUnits=deg  UpperLimitStiffness=1e4  UpperLimitStiffnessUnits=N*m/deg  UpperLimitDamping=10  UpperLimitDampingUnits=N*m/(deg/s)  UpperLimitTransitionRegionWidth=0.1  UpperLimitTransitionRegionWidthUnits=deg  PositionTargetSpecify=off  PositionTargetPriority=High  PositionTargetValue=0  PositionTargetValueUnits=deg  VelocityTargetSpecify=off  VelocityTargetPriority=High  VelocityTargetValue=0  VelocityTargetValueUnits=deg/s
  Rotational Multibody Interface : fl_lib/Mechanical/Multibody Interfaces/Rotational Multibody Interface  Commented=on
  Shaft : fl_lib/Mechanical/Rotational Elements/Inertia  Commented=on  inertia=0.000000001 kg*m^2  num_ports=foundation.enum.numPorts2.two  w_specify=off  w_priority=High  w=0 rad/s  w_nominal_specify=off  w_nominal_unit=rad/s  w_nominal_value=1  t_specify=off  t_priority=None  t=0 N*m  t_nominal_specify=off  t_nominal_unit=N*m  t_nominal_value=1
      settings: InternalSimscapePortConfiguration="{\"Bottom\":[],\"Left\":[{\"id\":\"I\",\"label\":\"\",\"type\":\"foundation.mechanical.rotational.rotational\"}],\"Right\":[{\"id\":\"J\",\"label\":\"\",\"type\":\"foundation.mechanical.rotational.rotational\"}],\"Top\":[]}"
  Simulink-PS Converter1 : nesl_utility/Simulink-PS Converter  Commented=on  PhysicalDomain=network_engine_domain  SubClassName=ps_input  LeftPortType=input  RightPortType=output  PseudoPeriodic=off  Frequencies=[]  NoiseDistribution=none  NoiseParameters=[]  Unit=1  AffineConversion=off  FilteringAndDerivatives=provide  SimscapeFilterOrder=1  InputFilterTimeConstant=0.001  UdotUserProvided=0
  Solver Configuration : nesl_utility/Solver Configuration  Commented=on  PhysicalDomain=network_engine_domain  SubClassName=solver  LeftPortType=input  RightPortType=generic  Tones=[]  Harmonics=[]  SimulateNoise=off  Profile=off  UseLocalSampling=off  EnableSwitchedLinearOptims=on  FrequencyDomain=off  UseCCode=off  RelTol=0.001  AbsTol=1e-06  MinStep=1e-09  ToWorkspace=off  RevertToSquareIcSolve=off  NumHomotopyIterations=100  PhasorMode=off  PhasorModeNumHarmonics=1  ConsistencySolver=NEWTON_FTOL  IndexReductionMethod=DerivativeReplacement  DoDC=off  ResidualTolerance=1e-09  ConsistencyTolSource=GLOBAL  ConsistencyAbsTol=0.001  ConsistencyRelTol=0.001  ConsistencyTolFactor=0.001  UseLocalSolver=on  LocalSolverChoice=NE_TRAPEZOIDAL_ADVANCER  ResolveIndetEquations=on  FunctionEvalNumThread=1  LocalSolverSampleTime=0.001  DoFixedCost=on  MaxNonlinIter=10  MaxModeIter=2  ComputeImpulses=off  ImpulseIterations=2  LinearAlgebra=Sparse  LinearAlgebraNumThread=0  EquationFormulation=NE_TIME_EF  DelaysMemoryBudget=1024  AutomaticFiltering=on  FilteringTimeConstant=0.001  PartitionStorageMethod=AS_NEEDED  PartitionMemoryBudget=1024  PartitionMethod=FAST  MultibodyUseLocalSolver=off  MultibodyLocalSolverChoice=ODE1  MultibodyLocalSolverSampleTime=0.001
  Conn1 : PMIOPort  Side=Left
  Conn2 : PMIOPort  Port=2  Side=Right
  Conn3 : PMIOPort  Port=3  Side=Left
  Conn4 : PMIOPort  Port=4  Side=Left
  Conn5 : PMIOPort  Port=5  Side=Right
  wires:
  "Prop spinning for show only LOL, put -0.0003 to show it spinning"/1 -> Simulink-PS Converter1/1
  connections:
  Simulink-PS Converter1/RConn1 -- Revolute Joint/LConn2
  Battery/LConn1 -- Motor/LConn1
  Rotational Multibody Interface/RConn2 -- Shaft/RConn1
  Motor/RConn2 -- Conn5/RConn1
  Mechanical Rotational Reference1/LConn1 -- Solver Configuration/RConn1 -- Motor/RConn3
  Motor/LConn3 -- Shaft/LConn1
  Battery/RConn1 -- Motor/RConn1 -- Electrical Reference/LConn1
  Revolute Joint/RConn2 -- Rotational Multibody Interface/RConn1
  Motor/LConn2 -- Conn4/RConn1
  Convection/LConn1 -- Battery/RConn2
  Mechanical Rotational Reference/LConn1 -- Rotational Multibody Interface/LConn2
  Convection/RConn1 -- Ambient Temperature/LConn1
  Battery/LConn2 -- PS Terminator/LConn1
  Rotational Multibody Interface/LConn1 -- Conn3/RConn1
  Revolute Joint/LConn1 -- Conn1/RConn1
  Revolute Joint/RConn1 -- Conn2/RConn1

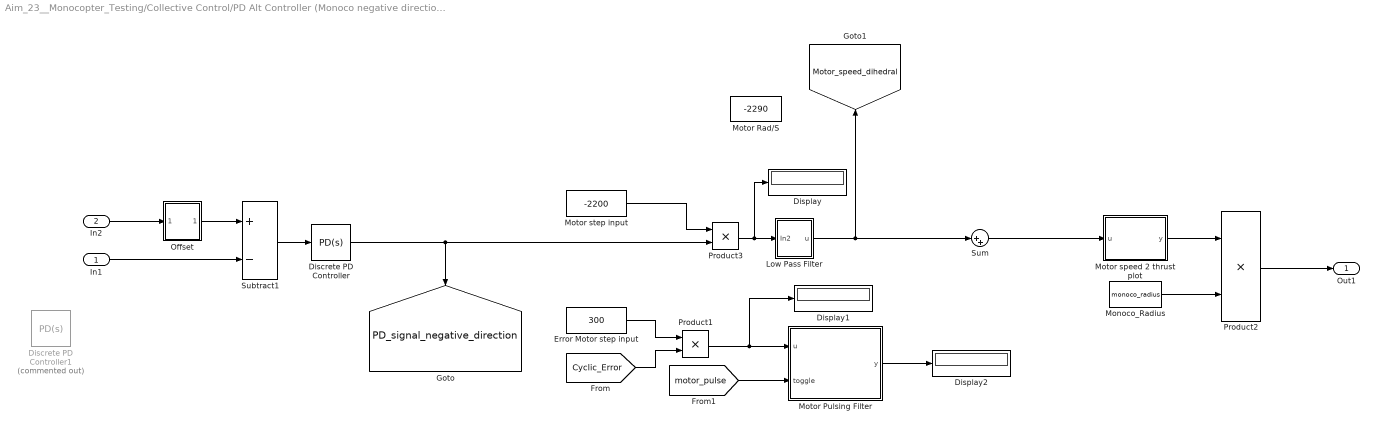
== system Aim_23__Monocopter_Testing/Collective Control/PD Alt Controller (Monoco negative direction counter clockwise) ==
  In1 : Inport
  In2 : Inport  Port=2
  Discrete PD Controller : slpidlib/PID Controller  Controller=PD  Form=Parallel  TimeDomain=Continuous-time  UseExternalTs=off  SampleTime=-1  IntegratorMethod=Forward Euler  FilterMethod=Forward Euler  ControllerParametersSource=internal  P=5.35  I=0.0  UseKiTs=off  D=1.25  N=filtD_motor  UseFilter=on  TunerSelectOption=Transfer Function Based (PID Tuner App)  InitialConditionSource=internal  InitialConditionForIntegrator=0  InitialConditionForFilter=0  DifferentiatorICPrevScaledInput=0  ExternalReset=none  TrackingMode=off  Kt=1  LimitOutput=off  SatLimitsSource=internal  UpperSaturationLimit=inf  LowerSaturationLimit=-inf  LinearizeAsGain=off  AntiWindupMode=none  Kb=1  LimitIntegrator=off  UpperIntegratorSaturationLimit=inf  LowerIntegratorSaturationLimit=-inf  POutMin=[]  POutMax=[]  IOutMin=[]  IOutMax=[]  DOutMin=[]  DOutMax=[]  NOutMin=[]  NOutMax=[]  SumOutMin=[]  SumOutMax=[]  SaturationOutMin=[]  SaturationOutMax=[]  PParamMin=[]  PParamMax=[]  IParamMin=[]  IParamMax=[]  DParamMin=[]  DParamMax=[]  NParamMin=[]  NParamMax=[]  KbParamMin=[]  KbParamMax=[]  KtParamMin=[]  KtParamMax=[]  KbOutMin=[]  KbOutMax=[]  KtOutMin=[]  KtOutMax=[]  IntegratorOutMin=[]  IntegratorOutMax=[]  FilterOutMin=[]  FilterOutMax=[]  SumI1OutMin=[]  SumI1OutMax=[]  SumI2OutMin=[]  SumI2OutMax=[]  SumI3OutMin=[]  SumI3OutMax=[]  SumI4OutMin=[]  SumI4OutMax=[]  SumDOutMin=[]  SumDOutMax=[]  DifferentiatorOutMin=[]  DifferentiatorOutMax=[]  FilterDiffOutCoefMin=[]  FilterDiffOutCoefMax=[]  ReciprocalOutMin=[]  ReciprocalOutMax=[]  SumDenOutMin=[]  SumDenOutMax=[]  SumNumOutMin=[]  SumNumOutMax=[]  DivideOutMin=[]  DivideOutMax=[]  UdiffTsProdOutMin=[]  UdiffTsProdOutMax=[]  NTsProdOutMin=[]  NTsProdOutMax=[]  UintegralTsProdOutMin=[]  UintegralTsProdOutMax=[]  UngainTsProdOutMin=[]  UngainTsProdOutMax=[]  ClampingZeroOutDataTypeStr=Inherit: Inherit via back propagation  ClampingZeroOutMin=[]  ClampingZeroOutMax=[]  FilterDenConstantOutDataTypeStr=Inherit: Inherit via back propagation  FilterDenConstantOutMin=[]  FilterDenConstantOutMax=[]  PCopyOutDataTypeStr=Inherit: Inherit via back propagation  PCopyOutMin=[]  PCopyOutMax=[]  NCopyOutDataTypeStr=Inherit: Inherit via back propagation  NCopyOutMin=[]  NCopyOutMax=[]  IntegratorContinuousStateAttributes=''  IntegratorStateMustResolveToSignalObject=off  IntegratorRTWStateStorageClass=Auto  FilterContinuousStateAttributes=''  FilterStateMustResolveToSignalObject=off  FilterRTWStateStorageClass=Auto  ParallelPVariant=InternalParameters  IdealPVariant=Disabled  IVariant=Disabled  DVariant=InternalParameters  IntegratorVariant=Disabled  SatVariant=Disabled  AWVariant=Disabled  PCopyVariant=Disabled  TRVariant=Disabled  FdbkBlocksVariant=Forward  IdealPFdbkVariant=Disabled  SatFdbkVariant=Disabled  DerivativeFilterVariant=ContFilter  NVariant=InternalParameters  NCopyVariant=Disabled  FilterICVariant=InternalICsFilter  IntegratorICVariant=Disabled  ExternalResetVariant=Disabled  TRSumVariant=Passthrough  SumFdbkVariant=Disabled  SumVariant=Sum_PD  TsampFilterVariant=InternalTs  TsampNgainVariant=Passthrough  TsampIntegralVariant=Disabled_SignalSpec  ExternalSaturationOutDataTypeStr=Inherit: Same as second input
      settings: LibrarySourceBlock=simulink/Discrete/Discrete PID Controller
  Discrete PD Controller1 : slpidlib/PID Controller  Commented=on  Controller=PD  Form=Parallel  TimeDomain=Continuous-time  UseExternalTs=off  SampleTime=-1  IntegratorMethod=Forward Euler  FilterMethod=Forward Euler  ControllerParametersSource=internal  P=5.35  I=0.0  UseKiTs=off  D=1.25  N=filtD_motor  UseFilter=on  TunerSelectOption=Transfer Function Based (PID Tuner App)  InitialConditionSource=internal  InitialConditionForIntegrator=0  InitialConditionForFilter=0  DifferentiatorICPrevScaledInput=0  ExternalReset=none  TrackingMode=off  Kt=1  LimitOutput=off  SatLimitsSource=internal  UpperSaturationLimit=inf  LowerSaturationLimit=-inf  LinearizeAsGain=off  AntiWindupMode=none  Kb=1  LimitIntegrator=off  UpperIntegratorSaturationLimit=inf  LowerIntegratorSaturationLimit=-inf  POutMin=[]  POutMax=[]  IOutMin=[]  IOutMax=[]  DOutMin=[]  DOutMax=[]  NOutMin=[]  NOutMax=[]  SumOutMin=[]  SumOutMax=[]  SaturationOutMin=[]  SaturationOutMax=[]  PParamMin=[]  PParamMax=[]  IParamMin=[]  IParamMax=[]  DParamMin=[]  DParamMax=[]  NParamMin=[]  NParamMax=[]  KbParamMin=[]  KbParamMax=[]  KtParamMin=[]  KtParamMax=[]  KbOutMin=[]  KbOutMax=[]  KtOutMin=[]  KtOutMax=[]  IntegratorOutMin=[]  IntegratorOutMax=[]  FilterOutMin=[]  FilterOutMax=[]  SumI1OutMin=[]  SumI1OutMax=[]  SumI2OutMin=[]  SumI2OutMax=[]  SumI3OutMin=[]  SumI3OutMax=[]  SumI4OutMin=[]  SumI4OutMax=[]  SumDOutMin=[]  SumDOutMax=[]  DifferentiatorOutMin=[]  DifferentiatorOutMax=[]  FilterDiffOutCoefMin=[]  FilterDiffOutCoefMax=[]  ReciprocalOutMin=[]  ReciprocalOutMax=[]  SumDenOutMin=[]  SumDenOutMax=[]  SumNumOutMin=[]  SumNumOutMax=[]  DivideOutMin=[]  DivideOutMax=[]  UdiffTsProdOutMin=[]  UdiffTsProdOutMax=[]  NTsProdOutMin=[]  NTsProdOutMax=[]  UintegralTsProdOutMin=[]  UintegralTsProdOutMax=[]  UngainTsProdOutMin=[]  UngainTsProdOutMax=[]  ClampingZeroOutDataTypeStr=Inherit: Inherit via back propagation  ClampingZeroOutMin=[]  ClampingZeroOutMax=[]  FilterDenConstantOutDataTypeStr=Inherit: Inherit via back propagation  FilterDenConstantOutMin=[]  FilterDenConstantOutMax=[]  PCopyOutDataTypeStr=Inherit: Inherit via back propagation  PCopyOutMin=[]  PCopyOutMax=[]  NCopyOutDataTypeStr=Inherit: Inherit via back propagation  NCopyOutMin=[]  NCopyOutMax=[]  IntegratorContinuousStateAttributes=''  IntegratorStateMustResolveToSignalObject=off  IntegratorRTWStateStorageClass=Auto  FilterContinuousStateAttributes=''  FilterStateMustResolveToSignalObject=off  FilterRTWStateStorageClass=Auto  ParallelPVariant=InternalParameters  IdealPVariant=Disabled  IVariant=Disabled  DVariant=InternalParameters  IntegratorVariant=Disabled  SatVariant=Disabled  AWVariant=Disabled  PCopyVariant=Disabled  TRVariant=Disabled  FdbkBlocksVariant=Forward  IdealPFdbkVariant=Disabled  SatFdbkVariant=Disabled  DerivativeFilterVariant=ContFilter  NVariant=InternalParameters  NCopyVariant=Disabled  FilterICVariant=InternalICsFilter  IntegratorICVariant=Disabled  ExternalResetVariant=Disabled  TRSumVariant=Passthrough  SumFdbkVariant=Disabled  SumVariant=Sum_PD  TsampFilterVariant=InternalTs  TsampNgainVariant=Passthrough  TsampIntegralVariant=Disabled_SignalSpec  ExternalSaturationOutDataTypeStr=Inherit: Same as second input
      settings: LibrarySourceBlock=simulink/Discrete/Discrete PID Controller
  Display : Display
  Display1 : Display
  Display2 : Display
  Error Motor step input : Constant  Value=300
  Low Pass Filter : Subsystem
  Monoco_Radius : Constant  Value=monoco_radius
  Motor Pulsing Filter : MATLAB Function  TreatAsAtomicUnit=on
  Motor Rad/S : Constant  Value=-2290
  Motor speed 2 thrust plot : MATLAB Function  TreatAsAtomicUnit=on
  Motor step input : Constant  Value=-2200
  Offset : Subsystem
  Product1 : Product
  Product2 : Product
  Product3 : Product
  Subtract1 : Sum  Inputs=+-
  Sum : Sum  Inputs=|++
  Out1 : Outport
  tag scope: Motor_speed_dihedral=global, PD_signal_negative_direction=global
  wires:
  Product3/1 -> Display/1, Low Pass Filter/1(In2)
  Motor speed 2 thrust plot/1(y) -> Product2/1
  In2/1 -> Offset/1(In2)
  Offset/1(Out1) -> Subtract1/1
  Subtract1/1 -> Discrete PD Controller/1
  Monoco_Radius/1 -> Product2/2
  Low Pass Filter/1(u) -> Sum/1, [Motor_speed_dihedral]
  Discrete PD Controller/1 -> Product3/2, [PD_signal_negative_direction]
  Motor step input/1 -> Product3/1
  Product2/1 -> Out1/1
  In1/1 -> Subtract1/2
  Product1/1 -> Motor Pulsing Filter/1(u), Display1/1
  Error Motor step input/1 -> Product1/1
  [Cyclic_Error] -> Product1/2
  [motor_pulse] -> Motor Pulsing Filter/2(toggle)
  Sum/1 -> Motor speed 2 thrust plot/1(u)
  Motor Pulsing Filter/1(y) -> Display2/1

== system Aim_23__Monocopter_Testing/Collective Control/PD Alt Controller (Monoco positve direction clockwise) ==
  In2 : Inport
  In1 : Inport  Port=2
  Discrete PD Controller : slpidlib/PID Controller  Controller=PD  Form=Parallel  TimeDomain=Continuous-time  UseExternalTs=off  SampleTime=-1  IntegratorMethod=Forward Euler  FilterMethod=Forward Euler  ControllerParametersSource=internal  P=5.35  I=0.0  UseKiTs=off  D=1.25  N=filtD_motor  UseFilter=on  TunerSelectOption=Transfer Function Based (PID Tuner App)  InitialConditionSource=internal  InitialConditionForIntegrator=0  InitialConditionForFilter=0  DifferentiatorICPrevScaledInput=0  ExternalReset=none  TrackingMode=off  Kt=1  LimitOutput=off  SatLimitsSource=internal  UpperSaturationLimit=inf  LowerSaturationLimit=-inf  LinearizeAsGain=off  AntiWindupMode=none  Kb=1  LimitIntegrator=off  UpperIntegratorSaturationLimit=inf  LowerIntegratorSaturationLimit=-inf  POutMin=[]  POutMax=[]  IOutMin=[]  IOutMax=[]  DOutMin=[]  DOutMax=[]  NOutMin=[]  NOutMax=[]  SumOutMin=[]  SumOutMax=[]  SaturationOutMin=[]  SaturationOutMax=[]  PParamMin=[]  PParamMax=[]  IParamMin=[]  IParamMax=[]  DParamMin=[]  DParamMax=[]  NParamMin=[]  NParamMax=[]  KbParamMin=[]  KbParamMax=[]  KtParamMin=[]  KtParamMax=[]  KbOutMin=[]  KbOutMax=[]  KtOutMin=[]  KtOutMax=[]  IntegratorOutMin=[]  IntegratorOutMax=[]  FilterOutMin=[]  FilterOutMax=[]  SumI1OutMin=[]  SumI1OutMax=[]  SumI2OutMin=[]  SumI2OutMax=[]  SumI3OutMin=[]  SumI3OutMax=[]  SumI4OutMin=[]  SumI4OutMax=[]  SumDOutMin=[]  SumDOutMax=[]  DifferentiatorOutMin=[]  DifferentiatorOutMax=[]  FilterDiffOutCoefMin=[]  FilterDiffOutCoefMax=[]  ReciprocalOutMin=[]  ReciprocalOutMax=[]  SumDenOutMin=[]  SumDenOutMax=[]  SumNumOutMin=[]  SumNumOutMax=[]  DivideOutMin=[]  DivideOutMax=[]  UdiffTsProdOutMin=[]  UdiffTsProdOutMax=[]  NTsProdOutMin=[]  NTsProdOutMax=[]  UintegralTsProdOutMin=[]  UintegralTsProdOutMax=[]  UngainTsProdOutMin=[]  UngainTsProdOutMax=[]  ClampingZeroOutDataTypeStr=Inherit: Inherit via back propagation  ClampingZeroOutMin=[]  ClampingZeroOutMax=[]  FilterDenConstantOutDataTypeStr=Inherit: Inherit via back propagation  FilterDenConstantOutMin=[]  FilterDenConstantOutMax=[]  PCopyOutDataTypeStr=Inherit: Inherit via back propagation  PCopyOutMin=[]  PCopyOutMax=[]  NCopyOutDataTypeStr=Inherit: Inherit via back propagation  NCopyOutMin=[]  NCopyOutMax=[]  IntegratorContinuousStateAttributes=''  IntegratorStateMustResolveToSignalObject=off  IntegratorRTWStateStorageClass=Auto  FilterContinuousStateAttributes=''  FilterStateMustResolveToSignalObject=off  FilterRTWStateStorageClass=Auto  ParallelPVariant=InternalParameters  IdealPVariant=Disabled  IVariant=Disabled  DVariant=InternalParameters  IntegratorVariant=Disabled  SatVariant=Disabled  AWVariant=Disabled  PCopyVariant=Disabled  TRVariant=Disabled  FdbkBlocksVariant=Forward  IdealPFdbkVariant=Disabled  SatFdbkVariant=Disabled  DerivativeFilterVariant=ContFilter  NVariant=InternalParameters  NCopyVariant=Disabled  FilterICVariant=InternalICsFilter  IntegratorICVariant=Disabled  ExternalResetVariant=Disabled  TRSumVariant=Passthrough  SumFdbkVariant=Disabled  SumVariant=Sum_PD  TsampFilterVariant=InternalTs  TsampNgainVariant=Passthrough  TsampIntegralVariant=Disabled_SignalSpec  ExternalSaturationOutDataTypeStr=Inherit: Same as second input
      settings: LibrarySourceBlock=simulink/Discrete/Discrete PID Controller
  Low Pass Filter : Subsystem
  Monoco_Radius : Constant  Value=monoco_radius
  Motor Rad/S : Constant  Value=2290
  Motor speed 2 thrust plot : MATLAB Function  TreatAsAtomicUnit=on
  Motor step input : Constant  Value=2300
  Offset : Subsystem
  Product2 : Product
  Product3 : Product
  Subtract1 : Sum  Inputs=+-
  Out1 : Outport
  tag scope: Motor_speed_anhedral=global, PD_signal_positive_direction=global
  wires:
  Product3/1 -> Low Pass Filter/1(In2)
  Motor speed 2 thrust plot/1(y) -> Product2/1
  In2/1 -> Offset/1(In2)
  Offset/1(Out1) -> Subtract1/1
  Subtract1/1 -> Discrete PD Controller/1
  Monoco_Radius/1 -> Product2/2
  Low Pass Filter/1(u) -> Motor speed 2 thrust plot/1(u), [Motor_speed_anhedral]
  Discrete PD Controller/1 -> Product3/2, [PD_signal_positive_direction]
  Motor step input/1 -> Product3/1
  Product2/1 -> Out1/1
  In1/1 -> Subtract1/2

== system Aim_23__Monocopter_Testing/Control Modules/Bang Bang Control ==
  In1 : Inport
  Desired RPS1 : Constant  Value=-0.02
  Desired RPS2 : Constant  Value=0
  If : If  IfExpression=u1 > 1
  If Action Subsystem : Subsystem  TreatAsAtomicUnit=on
  If Action Subsystem1 : Subsystem  TreatAsAtomicUnit=on
  Merge : Merge
  Zero-Order Hold : ZeroOrderHold  SampleTime=-1
  Out1 : Outport
  wires:
  If/1 -> If Action Subsystem1/Action
  Desired RPS1/1 -> Zero-Order Hold/1
  If/2 -> If Action Subsystem/Action
  Zero-Order Hold/1 -> If Action Subsystem/1(In1)
  If Action Subsystem/1(Out1) -> Merge/2
  Desired RPS2/1 -> If Action Subsystem1/1(In1)
  In1/1 -> If/1
  If Action Subsystem1/1(Out1) -> Merge/1
  Merge/1 -> Out1/1

== system Aim_23__Monocopter_Testing/Control Modules/Bang Bang Control Ideal ==
  In1 : Inport
  Desired RPS1 : Constant  Value=-0.01475
  Desired RPS2 : Constant  Value=-0.0145
  If : If  IfExpression=u1 > 1
  If Action Subsystem : Subsystem  TreatAsAtomicUnit=on
  If Action Subsystem1 : Subsystem  TreatAsAtomicUnit=on
  Merge : Merge
  Zero-Order Hold : ZeroOrderHold  SampleTime=-1
  Out1 : Outport
  wires:
  If/1 -> If Action Subsystem1/Action
  Desired RPS1/1 -> Zero-Order Hold/1
  If/2 -> If Action Subsystem/Action
  Zero-Order Hold/1 -> If Action Subsystem/1(In1)
  If Action Subsystem/1(Out1) -> Merge/2
  Desired RPS2/1 -> If Action Subsystem1/1(In1)
  In1/1 -> If/1
  If Action Subsystem1/1(Out1) -> Merge/1
  Merge/1 -> Out1/1

== system Aim_23__Monocopter_Testing/Control Modules/PID Ideal1 ==
  u : Inport
  Discrete PID Controller : slpidlib/PID Controller  Controller=PD  Form=Parallel  TimeDomain=Continuous-time  UseExternalTs=off  SampleTime=-1  IntegratorMethod=Forward Euler  FilterMethod=Forward Euler  ControllerParametersSource=internal  P=1  I=0  UseKiTs=off  D=0.9  N=filtD_motor  UseFilter=on  TunerSelectOption=Transfer Function Based (PID Tuner App)  InitialConditionSource=internal  InitialConditionForIntegrator=0  InitialConditionForFilter=0  DifferentiatorICPrevScaledInput=0  ExternalReset=none  TrackingMode=off  Kt=1  LimitOutput=on  SatLimitsSource=internal  UpperSaturationLimit=inf  LowerSaturationLimit=-inf  LinearizeAsGain=off  AntiWindupMode=none  Kb=1  LimitIntegrator=off  UpperIntegratorSaturationLimit=inf  LowerIntegratorSaturationLimit=-inf  POutMin=[]  POutMax=[]  IOutMin=[]  IOutMax=[]  DOutMin=[]  DOutMax=[]  NOutMin=[]  NOutMax=[]  SumOutMin=[]  SumOutMax=[]  SaturationOutMin=[]  SaturationOutMax=[]  PParamMin=[]  PParamMax=[]  IParamMin=[]  IParamMax=[]  DParamMin=[]  DParamMax=[]  NParamMin=[]  NParamMax=[]  KbParamMin=[]  KbParamMax=[]  KtParamMin=[]  KtParamMax=[]  KbOutMin=[]  KbOutMax=[]  KtOutMin=[]  KtOutMax=[]  IntegratorOutMin=[]  IntegratorOutMax=[]  FilterOutMin=[]  FilterOutMax=[]  SumI1OutMin=[]  SumI1OutMax=[]  SumI2OutMin=[]  SumI2OutMax=[]  SumI3OutMin=[]  SumI3OutMax=[]  SumI4OutMin=[]  SumI4OutMax=[]  SumDOutMin=[]  SumDOutMax=[]  DifferentiatorOutMin=[]  DifferentiatorOutMax=[]  FilterDiffOutCoefMin=[]  FilterDiffOutCoefMax=[]  ReciprocalOutMin=[]  ReciprocalOutMax=[]  SumDenOutMin=[]  SumDenOutMax=[]  SumNumOutMin=[]  SumNumOutMax=[]  DivideOutMin=[]  DivideOutMax=[]  UdiffTsProdOutMin=[]  UdiffTsProdOutMax=[]  NTsProdOutMin=[]  NTsProdOutMax=[]  UintegralTsProdOutMin=[]  UintegralTsProdOutMax=[]  UngainTsProdOutMin=[]  UngainTsProdOutMax=[]  ClampingZeroOutDataTypeStr=Inherit: Inherit via back propagation  ClampingZeroOutMin=[]  ClampingZeroOutMax=[]  FilterDenConstantOutDataTypeStr=Inherit: Inherit via back propagation  FilterDenConstantOutMin=[]  FilterDenConstantOutMax=[]  PCopyOutDataTypeStr=Inherit: Inherit via back propagation  PCopyOutMin=[]  PCopyOutMax=[]  NCopyOutDataTypeStr=Inherit: Inherit via back propagation  NCopyOutMin=[]  NCopyOutMax=[]  IntegratorContinuousStateAttributes=''  IntegratorStateMustResolveToSignalObject=off  IntegratorRTWStateStorageClass=Auto  FilterContinuousStateAttributes=''  FilterStateMustResolveToSignalObject=off  FilterRTWStateStorageClass=Auto  ParallelPVariant=InternalParameters  IdealPVariant=Disabled  IVariant=Disabled  DVariant=InternalParameters  IntegratorVariant=Disabled  SatVariant=Enabled  AWVariant=Disabled  PCopyVariant=Disabled  TRVariant=Disabled  FdbkBlocksVariant=Forward  IdealPFdbkVariant=Disabled  SatFdbkVariant=Disabled  DerivativeFilterVariant=ContFilter  NVariant=InternalParameters  NCopyVariant=Disabled  FilterICVariant=InternalICsFilter  IntegratorICVariant=Disabled  ExternalResetVariant=Disabled  TRSumVariant=Passthrough  SumFdbkVariant=Disabled  SumVariant=Sum_PD  TsampFilterVariant=InternalTs  TsampNgainVariant=Passthrough  TsampIntegralVariant=Disabled_SignalSpec  ExternalSaturationOutDataTypeStr=Inherit: Same as second input
      settings: LibrarySourceBlock=simulink/Discrete/Discrete PID Controller
  Motor Control Input : Constant  Value=0.03
  Product : Product
  Wrap To Zero2 : simulink/Discontinuities/Wrap To Zero  Threshold=0
  Y : Outport
  wires:
  Motor Control Input/1 -> Product/1
  Discrete PID Controller/1 -> Product/2
  u/1 -> Discrete PID Controller/1
  Wrap To Zero2/1 -> Y/1
  Product/1 -> Wrap To Zero2/1
